simulink model "myo_sfun_two_myo"  (R2013a)
settings: Solver=ode3  StartTime=0.0  StopTime=inf  FixedStep=0.04  RelTol=1e-3
libraries: rtwinlib x1, myo_lib x1
settings Model: Creator=Mark Tomaszewski  LastModifiedBy=marktoma
settings GRTTargetCC: ExtMode=on

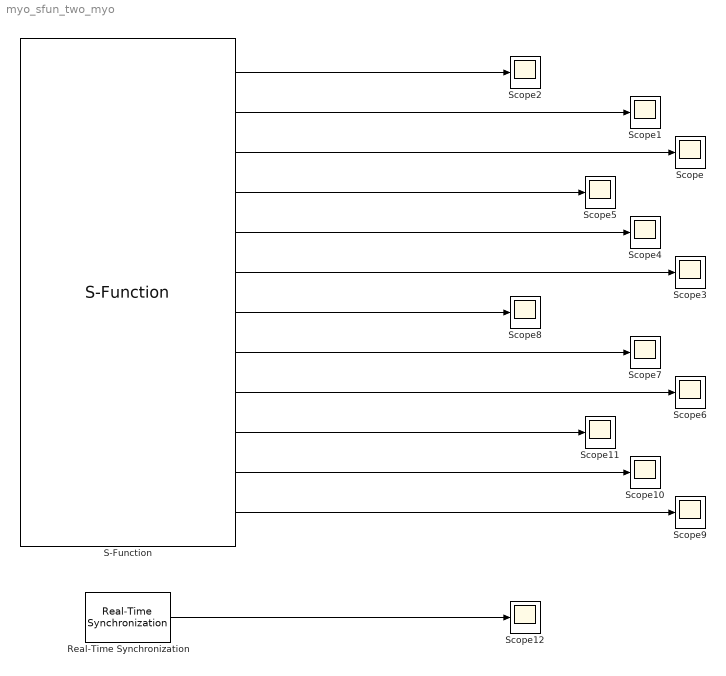
== system myo_sfun_two_myo ==
  Real-Time Synchronization : rtwinlib/Real-Time Synchronization  SampleTime=0.04  MaxMissedTicks=200  ShowMissedTicks=on  YieldWhenWaiting=off
  S-Function : myo_lib/S-Function  emgEnabled=0  countMyos=2
  Scope{,1..12} (13 alike) : Scope
      Scope1 settings: YMin=-750  YMax=1750
      Scope10 settings: SaveName=ScopeData6
      Scope11 settings: SaveName=ScopeData7
      Scope12 settings: SaveName=ScopeData12
      Scope2 settings: YMin=-0.5  YMax=1  SaveName=ScopeData2
      Scope3 settings: SaveName=ScopeData3
      Scope4 settings: SaveName=ScopeData4
      Scope5 settings: SaveName=ScopeData5
      Scope6 settings: SaveName=ScopeData8
      Scope7 settings: YMin=-750  YMax=1750  SaveName=ScopeData9
      Scope8 settings: YMin=-0.5  YMax=1  SaveName=ScopeData10
      Scope9 settings: SaveName=ScopeData11
  wires:
  S-Function/1 -> Scope2/1
  S-Function/2 -> Scope1/1
  S-Function/3 -> Scope/1
  S-Function/4 -> Scope5/1
  S-Function/5 -> Scope4/1
  S-Function/6 -> Scope3/1
  S-Function/7 -> Scope8/1
  S-Function/8 -> Scope7/1
  S-Function/9 -> Scope6/1
  S-Function/10 -> Scope11/1
  S-Function/11 -> Scope10/1
  S-Function/12 -> Scope9/1
  Real-Time Synchronization/1 -> Scope12/1
